simulink model "phi_ref"  (R2024b)
settings: Solver=FixedStepAuto  StartTime=0.0  StopTime=10.0  RelTol=1e-3
undefined symbols (not defined in the file): a, b, Ku
libraries: simulink x1
settings Model: Creator=marti  LastModifiedBy=marti

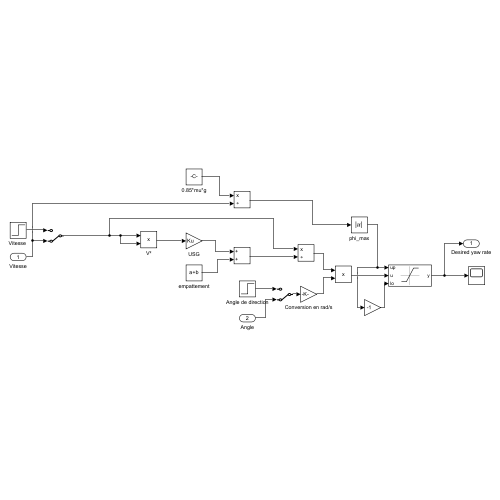
[thumbnail: Simulink's stored preview of the top-level diagram]
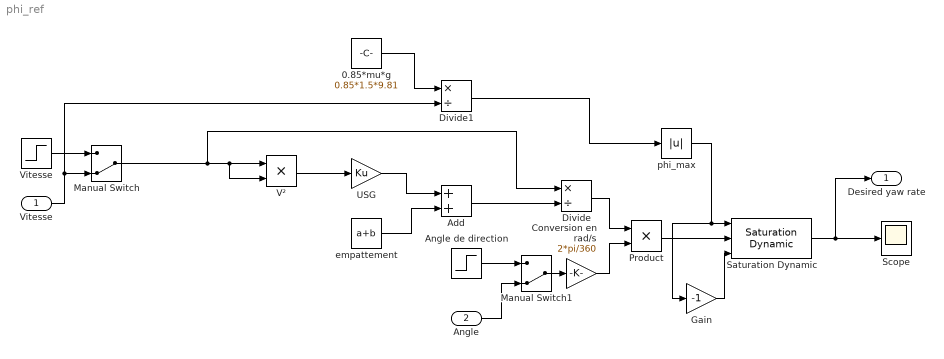
== system phi_ref ==
  Vitesse : Inport
  Angle : Inport  Port=2
  0.85*mu*g : Constant  Value=0.85*1.5*9.81
  Add : Sum
  Angle de direction : Step  Time=2  After=10  SampleTime=0
  Conversion en rad/s : Gain  Gain=2*pi/360
  Divide : Product  Inputs=*/
  Divide1 : Product  Inputs=*/
  Gain : Gain  Gain=-1
  Manual Switch : ManualSwitch  CurrentSetting=0
  Manual Switch1 : ManualSwitch  CurrentSetting=0
  Product : Product
  Saturation Dynamic : simulink/Discontinuities/Saturation Dynamic  OutMin=[]  OutMax=[]  OutDataTypeStr=Inherit: Same as second input  OutDataType=fixdt(1, 16)  OutScaling=2^-10  DoSatur=off
  Scope : Scope
  USG : Gain  Gain=Ku
  "Vitesse " : Step  After=20  SampleTime=0
  V² : Product
  empattement : Constant  Value=a+b
  phi_max : Abs  SaturateOnIntegerOverflow=off
  Desired yaw rate : Outport
  wires:
  Manual Switch/1 -> Divide/1, V²/2, V²/1
  V²/1 -> USG/1
  USG/1 -> Add/1
  empattement/1 -> Add/2
  Add/1 -> Divide/2
  Divide/1 -> Product/1
  Conversion en rad/s/1 -> Product/2
  Saturation Dynamic/1 -> Desired yaw rate/1, Scope/1
  Vitesse/1 -> Divide1/2, Manual Switch/2
  "Vitesse "/1 -> Manual Switch/1
  Manual Switch1/1 -> Conversion en rad/s/1
  Angle de direction/1 -> Manual Switch1/1
  Angle/1 -> Manual Switch1/2
  0.85*mu*g/1 -> Divide1/1
  Divide1/1 -> phi_max/1
  Product/1 -> Saturation Dynamic/2
  phi_max/1 -> Gain/1, Saturation Dynamic/1
  Gain/1 -> Saturation Dynamic/3
